simulink model "modLoad_1"  (R2019b)
settings: Solver=VariableStepAuto  StartTime=0.0  StopTime=300.0  RelTol=1e-3
values from neighbouring files (symbols this model uses):
  c = 2    [exer.m]
  inertia = 100    [exer.m]
  torqueDriveSet = 314    [exer.m]
  tStep = 0    [exer.m]
settings Model: Creator=edxu96  LastModifiedBy=edxu96

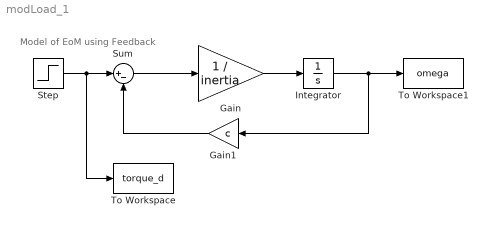
== system modLoad_1 ==
  note: Model of EoM using Feedback
  Gain : Gain  Gain=1 / inertia
  Gain1 : Gain  Gain=c
  Integrator : Integrator  InitialCondition=torqueDriveSet  ContinuousStateAttributes='omega'
  Step : Step  Time=tStep  After=200  SampleTime=0
  Sum : Sum  Inputs=|+-
  To Workspace : ToWorkspace  VariableName=torque_d  SaveFormat=Structure With Time  SampleTime=-1
  To Workspace1 : ToWorkspace  VariableName=omega  SaveFormat=Structure With Time  SampleTime=-1
  wires:
  Gain/1 -> Integrator/1
  Step/1 -> Sum/1, To Workspace/1
  Gain1/1 -> Sum/2
  Integrator/1 -> To Workspace1/1, Gain1/1
  Sum/1 -> Gain/1
